simulink model "I_controller"  (R2018a)
settings: Solver=VariableStepAuto  StartTime=0.0  StopTime=500  RelTol=1e-3
settings Model: Creator=mjb15180  LastModifiedBy=mjb15180

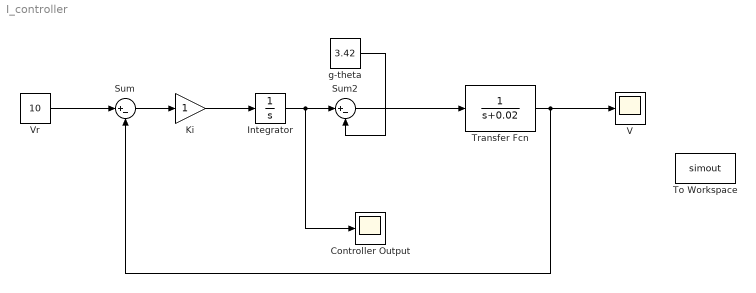
== system I_controller ==
  Controller Output : Scope
  Integrator : Integrator  InitialCondition=1
  Ki : Gain
  Sum : Sum  Inputs=|+-
  Sum2 : Sum  Inputs=|+-
  To Workspace : ToWorkspace  VariableName=simout  SaveFormat=Timeseries  SampleTime=-1
  Transfer Fcn : TransferFcn  Denominator=[1 0.02]
  V : Scope
  Vr : Constant  Value=10
  g-theta : Constant  Value=3.42
  wires:
  Sum2/1 -> Transfer Fcn/1
  Transfer Fcn/1 -> Sum/2, V/1
  Integrator/1 -> Controller Output/1, Sum2/1
  g-theta/1 -> Sum2/2
  Sum/1 -> Ki/1
  Ki/1 -> Integrator/1
  Vr/1 -> Sum/1
